simulink model "AIES_3R_2015b"  (R2015b)
settings: Solver=VariableStepAuto  SolverMode=SingleTasking  StartTime=0.0  StopTime=11  RelTol=1e-3
settings Model: Creator=Javad  LastModifiedBy=Armin
settings DataIOCC: LimitDataPoints=off  ReturnWorkspaceOutputs=on
settings DebuggingCC: AllowSymbolicDim=on  SFUnexpectedBacktrackingDiag=error  SFNoUnconditionalDefaultTransitionDiag=error
settings ModelReferenceCC: PropagateSignalLabelsOutOfModel=on
settings SFSimCC: SimUseLocalCustomCode=on
settings RTWCC: RTWUseLocalCustomCode=on
settings GRTTargetCC: TargetLangStandard=C99 (ISO)
settings ConfigComp: CovMetricSettings=dwe  CovSaveCumulativeToWorkspaceVar=off  CovSaveSingleToWorkspaceVar=off  CovModelRefEnable=Off  CovExternalEMLEnable=on

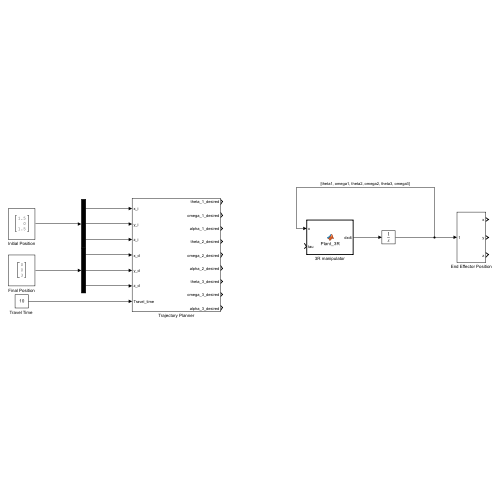
[thumbnail: Simulink's stored preview of the top-level diagram]
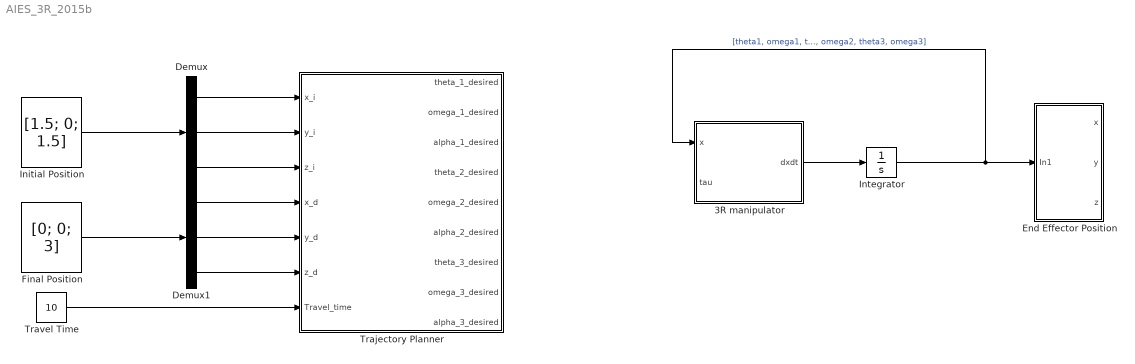
== system AIES_3R_2015b ==
  3R manipulator : MATLAB Function  TreatAsAtomicUnit=on
  Demux : Demux  Outputs=3
  Demux1 : Demux  Outputs=3
  End Effector Position : Subsystem
  Final Position : Constant  Value=[0; 0; 3]  VectorParams1D=off
  Initial Position : Constant  Value=[1.5; 0; 1.5]  VectorParams1D=off
  Integrator : Integrator
  Trajectory Planner : Subsystem
  "Travel Time " : Constant  Value=10
  wires:
  Initial Position/1 -> Demux/1
  Demux/1 -> Trajectory Planner/1(x_i)
  Demux/2 -> Trajectory Planner/2(y_i)
  Demux/3 -> Trajectory Planner/3(z_i)
  "Travel Time "/1 -> Trajectory Planner/7(Travel_time)
  Final Position/1 -> Demux1/1
  Demux1/1 -> Trajectory Planner/4(x_d)
  Demux1/2 -> Trajectory Planner/5(y_d)
  Demux1/3 -> Trajectory Planner/6(z_d)
  3R manipulator/1(dxdt) -> Integrator/1
  Integrator/1 -> End Effector Position/1(In1), 3R manipulator/1(x)  "[theta1, omega1, theta2, omega2, theta3, omega3]"

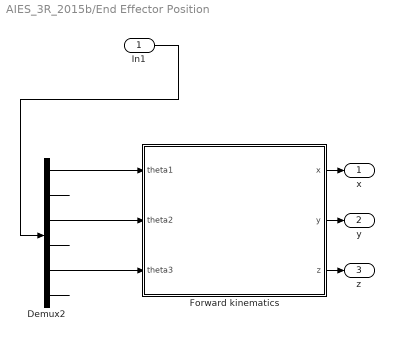
== system AIES_3R_2015b/End Effector Position ==
  In1 : Inport
  Demux2 : Demux  Outputs=6
  Forward kinematics : MATLAB Function  TreatAsAtomicUnit=on
  x : Outport
  y : Outport  Port=2
  z : Outport  Port=3
  wires:
  Demux2/1 -> Forward kinematics/1(theta1)
  In1/1 -> Demux2/1
  Forward kinematics/2(y) -> y/1
  Demux2/3 -> Forward kinematics/2(theta2)
  Demux2/4 -> ?
  Forward kinematics/3(z) -> z/1
  Forward kinematics/1(x) -> x/1
  Demux2/2 -> ?
  Demux2/5 -> Forward kinematics/3(theta3)
  Demux2/6 -> ?

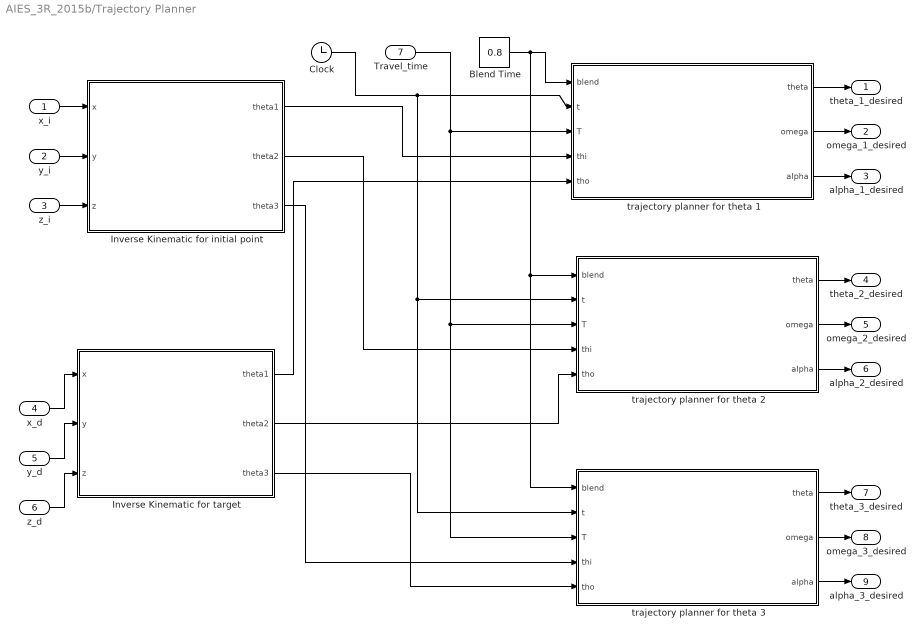
== system AIES_3R_2015b/Trajectory Planner ==
  x_i : Inport
  y_i : Inport  Port=2
  z_i : Inport  Port=3
  x_d : Inport  Port=4
  y_d : Inport  Port=5
  z_d : Inport  Port=6
  Travel_time : Inport  Port=7
  Blend Time : Constant  Value=0.8
  Clock : Clock
  Inverse Kinematic for initial point : MATLAB Function  TreatAsAtomicUnit=on
  Inverse Kinematic for target : MATLAB Function  TreatAsAtomicUnit=on
  trajectory planner for theta 1 : MATLAB Function  TreatAsAtomicUnit=on
  trajectory planner for theta 2 : MATLAB Function  TreatAsAtomicUnit=on
  trajectory planner for theta 3 : MATLAB Function  TreatAsAtomicUnit=on
  theta_1_desired : Outport
  omega_1_desired : Outport  Port=2
  alpha_1_desired : Outport  Port=3
  theta_2_desired : Outport  Port=4
  omega_2_desired : Outport  Port=5
  alpha_2_desired : Outport  Port=6
  theta_3_desired : Outport  Port=7
  omega_3_desired : Outport  Port=8
  alpha_3_desired : Outport  Port=9
  wires:
  trajectory planner for theta 1/2(omega) -> omega_1_desired/1
  y_i/1 -> Inverse Kinematic for initial point/2(y)
  trajectory planner for theta 1/1(theta) -> theta_1_desired/1
  Inverse Kinematic for initial point/1(theta1) -> trajectory planner for theta 1/4(thi)
  Inverse Kinematic for target/1(theta1) -> trajectory planner for theta 1/5(tho)
  trajectory planner for theta 1/3(alpha) -> alpha_1_desired/1
  x_i/1 -> Inverse Kinematic for initial point/1(x)
  z_i/1 -> Inverse Kinematic for initial point/3(z)
  Inverse Kinematic for initial point/2(theta2) -> trajectory planner for theta 2/4(thi)
  trajectory planner for theta 2/3(alpha) -> alpha_2_desired/1
  trajectory planner for theta 2/2(omega) -> omega_2_desired/1
  trajectory planner for theta 2/1(theta) -> theta_2_desired/1
  Inverse Kinematic for target/2(theta2) -> trajectory planner for theta 2/5(tho)
  Clock/1 -> trajectory planner for theta 1/2(t), trajectory planner for theta 3/2(t), trajectory planner for theta 2/2(t)
  Inverse Kinematic for target/3(theta3) -> trajectory planner for theta 3/5(tho)
  trajectory planner for theta 3/1(theta) -> theta_3_desired/1
  Inverse Kinematic for initial point/3(theta3) -> trajectory planner for theta 3/4(thi)
  Travel_time/1 -> trajectory planner for theta 1/3(T), trajectory planner for theta 2/3(T), trajectory planner for theta 3/3(T)
  trajectory planner for theta 3/2(omega) -> omega_3_desired/1
  Blend Time/1 -> trajectory planner for theta 2/1(blend), trajectory planner for theta 3/1(blend), trajectory planner for theta 1/1(blend)
  trajectory planner for theta 3/3(alpha) -> alpha_3_desired/1
  z_d/1 -> Inverse Kinematic for target/3(z)
  x_d/1 -> Inverse Kinematic for target/1(x)
  y_d/1 -> Inverse Kinematic for target/2(y)

== matlab function AIES_3R_2015b/Trajectory Planner/Inverse Kinematic for initial point ==
  data: x input; theta1 output; y input; z input; theta2 output; theta3 output
function [theta1, theta2, theta3] = inverse_kinematic(x, y, z)

L1=1.5; L2=0.8; L3=0.7;
theta1 = atan2(y, x);
theta3 = acos((x^2+y^2+(z-L1)^2-L2^2-L3^2)/(2*L2*L3));
phi = atan2(L3*sin(theta3), L3*cos(theta3)+L2);
theta2 = asin((z-L1)*cos(phi)/(L3*cos(theta3)+L2))-phi;

end

== matlab function AIES_3R_2015b/3R manipulator ==
  data: x input size=[6,1]; dxdt output size=[6,1]; tau input size=[3,1]

function dxdt = Plant_3R (x, tau)
th1 = x(1);
th1_d = x(2);
th2 = x(3);
th2_d = x(4);
th3 = x(5);
th3_d = x(6);
dxdt = zeros(6,1);
dxdt(1) = th1_d;
dxdt(2) = (2.4e+3*tau(1)-670.0*th1_d*th2_d*sin(th3)+...
    290.0*th1_d*th2_d*sin(2.0*th2+2.0*th3)+...
    290.0*th1_d*th3_d*sin(2.0*th2+2.0*th3)+...
    670.0*th1_d*th2_d*sin(2.0*th2+th3)+...
    380.0*th1_d*th2_d*sin(2.0*th2))/(340.0*cos(2.0*th2+th3)+...
    190.0*cos(2.0*th2)+340.0*cos(th3)+150.0*cos(2.0*th2+2.0*th3)+1.5e+3);
dxdt(3) = th2_d;
dxdt(4) = -0.38*sin(2.0*th2)*th1_d^2-18.0*cos(th2)+4.7*tau(2)-4.7*tau(3);
dxdt(5) = th3_d;
dxdt(6) = 16.0*cos(th2-1.0*th3)+85.0*cos(th2+th3)+18.0*cos(th2)-...
    0.86*th1_d^2*sin(th3)-1.7*th2_d^2*sin(th3)+...
    0.32*th1_d^2*sin(2.0*th2-1.0*th3)-...
    0.38*th1_d^2*sin(2.0*th2+2.0*th3)-...
    0.54*th1_d^2*sin(2.0*th2+th3)+0.38*th1_d^2*sin(2.0*th2)+...
    11.0*tau(3)-4.7*tau(2);

end

== matlab function AIES_3R_2015b/Trajectory Planner/trajectory planner for theta 1 ==
  data: blend input; t input; theta output; T input; thi input; tho input; omega output; alpha output
function [theta, omega, alpha] = trajectory_planner(blend, t, T, thi, tho)
%t is the current time
%T is the toal time of the movement. 
%thi is the initial angle
%tho is the target angle
% blend = 1;

V_max = (tho-thi)/(T-blend);
a = V_max/blend;

if t<=blend
    alpha = a;
    omega = a*t;
    theta = 1/2*a*t.^2+thi;
elseif t<=(T-blend)
    alpha = 0;
    omega = V_max;
    theta = 1/2*a*blend^2+thi+V_max.*(t-blend);
elseif t<=(T)
    alpha = -a;
    omega = V_max-a.*(t-(T-blend));
    theta = -1/2*a.*(t-(T-blend)).^2+V_max*(t-(T-blend))+1/2*a*blend^2+thi+...
        V_max*(T-2*blend);
else
    alpha = 0;
    omega = 0;
    theta = tho;
end
    
end

== matlab function AIES_3R_2015b/Trajectory Planner/trajectory planner for theta 2 ==
  data: blend input; t input; theta output; T input; thi input; tho input; omega output; alpha output
function [theta, omega, alpha] = trajectory_planner(blend, t, T, thi, tho)
%t is the current time
%T is the toal time of the movement. 
%thi is the initial angle
%tho is the target angle
% blend = 1;

V_max = (tho-thi)/(T-blend);
a = V_max/blend;

if t<=blend
    alpha = a;
    omega = a*t;
    theta = 1/2*a*t.^2+thi;
elseif t<=(T-blend)
    alpha = 0;
    omega = V_max;
    theta = 1/2*a*blend^2+thi+V_max.*(t-blend);
elseif t<=(T)
    alpha = -a;
    omega = V_max-a.*(t-(T-blend));
    theta = -1/2*a.*(t-(T-blend)).^2+V_max*(t-(T-blend))+1/2*a*blend^2+thi+...
        V_max*(T-2*blend);
else
    alpha = 0;
    omega = 0;
    theta = tho;
end
    
end

== matlab function AIES_3R_2015b/Trajectory Planner/trajectory planner for theta 3 ==
  data: blend input; t input; theta output; T input; thi input; tho input; omega output; alpha output
function [theta, omega, alpha] = trajectory_planner(blend, t, T, thi, tho)
%t is the current time
%T is the toal time of the movement. 
%thi is the initial angle
%tho is the target angle
% blend = 1;

V_max = (tho-thi)/(T-blend);
a = V_max/blend;

if t<=blend
    alpha = a;
    omega = a*t;
    theta = 1/2*a*t.^2+thi;
elseif t<=(T-blend)
    alpha = 0;
    omega = V_max;
    theta = 1/2*a*blend^2+thi+V_max.*(t-blend);
elseif t<=(T)
    alpha = -a;
    omega = V_max-a.*(t-(T-blend));
    theta = -1/2*a.*(t-(T-blend)).^2+V_max*(t-(T-blend))+1/2*a*blend^2+thi+...
        V_max*(T-2*blend);
else
    alpha = 0;
    omega = 0;
    theta = tho;
end
    
end

== matlab function AIES_3R_2015b/Trajectory Planner/Inverse Kinematic for target ==
  data: x input; theta1 output; y input; z input; theta2 output; theta3 output
function [theta1, theta2, theta3] = inverse_kinematic(x, y, z)

L1=1.5; L2=0.8; L3=0.7;
theta1 = atan2(y, x);
theta3 = acos((x^2+y^2+(z-L1)^2-L2^2-L3^2)/(2*L2*L3));
phi = atan2(L3*sin(theta3), L3*cos(theta3)+L2);
theta2 = asin((z-L1)*cos(phi)/(L3*cos(theta3)+L2))-phi;

end

== matlab function AIES_3R_2015b/End Effector Position/Forward kinematics ==
  data: x output; theta1 input; y output; theta2 input; theta3 input; z output
function [x, y, z] = fcn(theta1, theta2, theta3)

L1=1.5; L2=0.8; L3=0.7;

T_01 = [cos(theta1) -sin(theta1) 0  0;
        sin(theta1)  cos(theta1) 0  0;
        0            0           1  L1;
        0            0           0  1];
    
T_12 = [cos(theta2) -sin(theta2) 0  0;
        0            0          -1  0;
        sin(theta2)  cos(theta2) 0  0;
        0            0           0  1];
    
T_23 = [cos(theta3) -sin(theta3) 0  L2;
        sin(theta3)  cos(theta3) 0  0;
        0            0           1  0;
        0            0           0  1];

T_34 = [1            0           0  L3;
        0            1           0  0;
        0            0           1  0;
        0            0           0  1];
    
T_04 = (T_01*T_12*T_23*T_34);

x = T_04(1,4);
y = T_04(2,4);
z = T_04(3,4);
end
